simulink model "modulators"  (R2014a)
settings: Solver=ode1  StartTime=0.0  StopTime=Tsim  FixedStep=Ts  RelTol=1e-3
InitFcn:
  | GlobalParam;
undefined symbols (not defined in the file): fm, nc, tetaa, tetab, tetac, Tm, vcrls, Vs, we
libraries: simulink x36
settings Model: Creator=Leocompa  LastModifiedBy=Leocompa

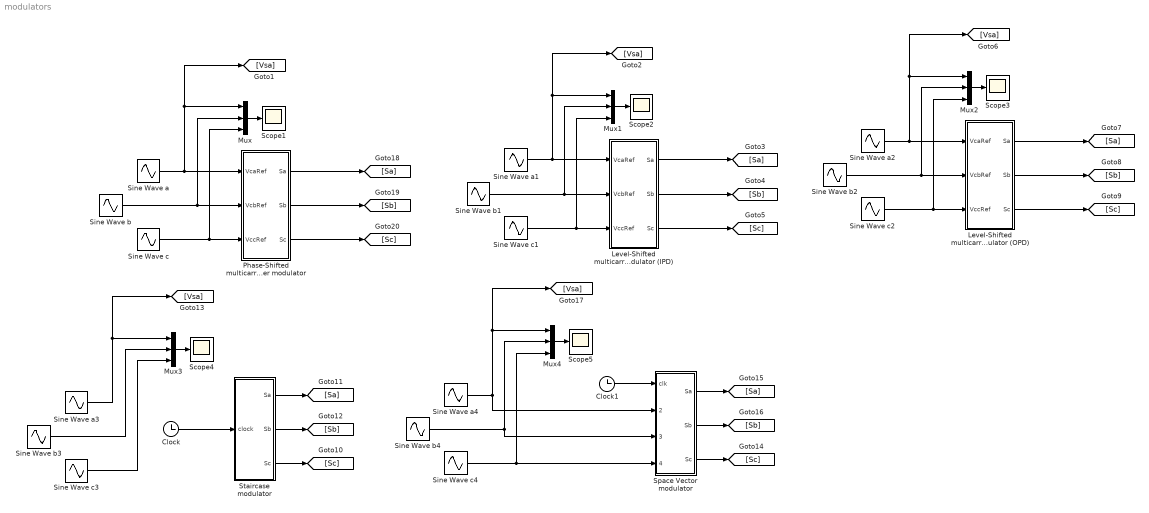
== system modulators ==
  Clock : Clock
  Clock1 : Clock
  Level-Shifted multicarrier modulator (IPD) : Subsystem
  Level-Shifted multicarrier modulator (OPD) : Subsystem
  Mux{,1..4} (5 alike) : Mux  Inputs=3
  Phase-Shifted multicarrier modulator : Subsystem
  Scope{1..5} (5 alike) : Scope
      Scope1 settings: YMin=-2500  YMax=37500  SaveName=vca1
      Scope2 settings: YMin=-2500  YMax=37500  SaveName=vca
      Scope3 settings: YMin=-2500  YMax=37500  SaveName=vca2
      Scope4 settings: YMin=-2500  YMax=37500  SaveName=vca3
      Scope5 settings: YMin=-2500  YMax=37500  SaveName=vca4
  Sine Wave a : Sin  Amplitude=Vs  Frequency=we  Phase=tetaa  SampleTime=0
  Sine Wave a1 : Sin  Amplitude=Vs  Frequency=we  SampleTime=0
  Sine Wave a2 : Sin  Amplitude=Vs  Frequency=we  SampleTime=0
  Sine Wave a3 : Sin  Amplitude=Vs  Frequency=we  Phase=tetaa  SampleTime=0
  Sine Wave a4 : Sin  Amplitude=Vs  Frequency=we  Phase=tetaa  SampleTime=0
  Sine Wave b{,1..4} (5 alike) : Sin  Amplitude=Vs  Frequency=we  Phase=tetab*pi/180  SampleTime=0
  Sine Wave c{,1..4} (5 alike) : Sin  Amplitude=Vs  Frequency=we  Phase=tetac*pi/180  SampleTime=0
  Space Vector modulator : Subsystem
  Staircase modulator : Subsystem
  wires:
  Phase-Shifted multicarrier modulator/1(Sa) -> [Sa]
  Phase-Shifted multicarrier modulator/2(Sb) -> [Sb]
  Phase-Shifted multicarrier modulator/3(Sc) -> [Sc]
  Sine Wave a/1 -> [Vsa], Mux/1, Phase-Shifted multicarrier modulator/1(VcaRef)
  Sine Wave b/1 -> Mux/2, Phase-Shifted multicarrier modulator/2(VcbRef)
  Sine Wave c/1 -> Mux/3, Phase-Shifted multicarrier modulator/3(VccRef)
  Mux/1 -> Scope1/1
  Level-Shifted multicarrier modulator (IPD)/1(Sa) -> [Sa]
  Level-Shifted multicarrier modulator (IPD)/2(Sb) -> [Sb]
  Level-Shifted multicarrier modulator (IPD)/3(Sc) -> [Sc]
  Sine Wave a1/1 -> [Vsa], Mux1/1, Level-Shifted multicarrier modulator (IPD)/1(VcaRef)
  Sine Wave b1/1 -> Mux1/2, Level-Shifted multicarrier modulator (IPD)/2(VcbRef)
  Sine Wave c1/1 -> Mux1/3, Level-Shifted multicarrier modulator (IPD)/3(VccRef)
  Mux1/1 -> Scope2/1
  Level-Shifted multicarrier modulator (OPD)/1(Sa) -> [Sa]
  Level-Shifted multicarrier modulator (OPD)/2(Sb) -> [Sb]
  Level-Shifted multicarrier modulator (OPD)/3(Sc) -> [Sc]
  Sine Wave a2/1 -> [Vsa], Mux2/1, Level-Shifted multicarrier modulator (OPD)/1(VcaRef)
  Sine Wave b2/1 -> Mux2/2, Level-Shifted multicarrier modulator (OPD)/2(VcbRef)
  Sine Wave c2/1 -> Mux2/3, Level-Shifted multicarrier modulator (OPD)/3(VccRef)
  Mux2/1 -> Scope3/1
  Sine Wave a3/1 -> [Vsa], Mux3/1
  Sine Wave b3/1 -> Mux3/2
  Sine Wave c3/1 -> Mux3/3
  Mux3/1 -> Scope4/1
  Clock/1 -> Staircase modulator/1(clock)
  Staircase modulator/3(Sc) -> [Sc]
  Staircase modulator/2(Sb) -> [Sb]
  Staircase modulator/1(Sa) -> [Sa]
  Sine Wave a4/1 -> Space Vector modulator/2(vca ref), [Vsa], Mux4/1
  Sine Wave b4/1 -> Mux4/2, Space Vector modulator/3(vcb ref1)
  Sine Wave c4/1 -> Mux4/3, Space Vector modulator/4(vcc ref2)
  Mux4/1 -> Scope5/1
  Clock1/1 -> Space Vector modulator/1(clk)
  Space Vector modulator/3(Sc) -> [Sc]
  Space Vector modulator/2(Sb) -> [Sb]
  Space Vector modulator/1(Sa) -> [Sa]

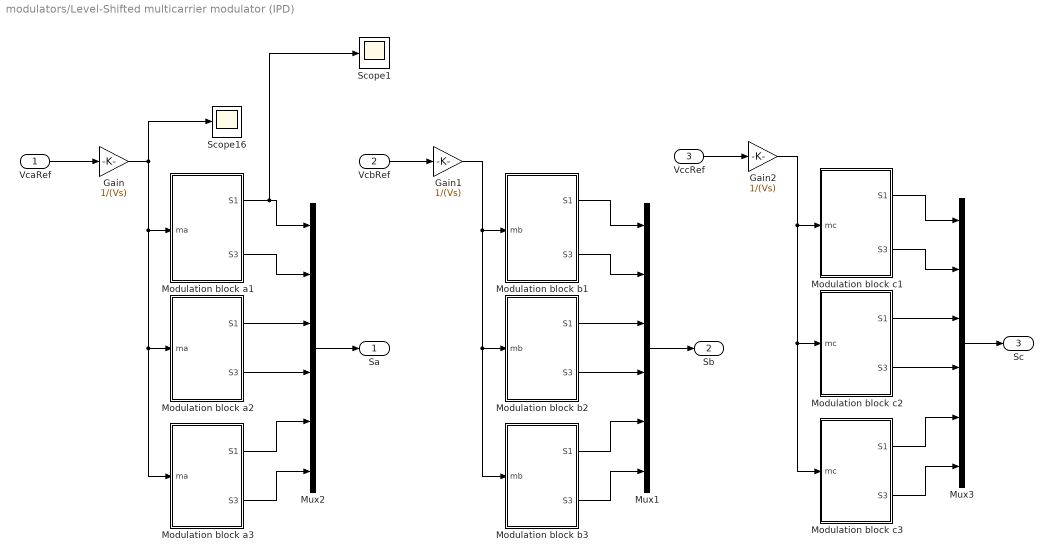
== system modulators/Level-Shifted multicarrier modulator (IPD) ==
  VcaRef : Inport
  VcbRef : Inport  Port=2
  VccRef : Inport  Port=3
  Gain : Gain  Gain=1/(Vs)
  Gain1 : Gain  Gain=1/(Vs)
  Gain2 : Gain  Gain=1/(Vs)
  Modulation block a1 : Subsystem
  Modulation block a2 : Subsystem
  Modulation block a3 : Subsystem
  Modulation block b1 : Subsystem
  Modulation block b2 : Subsystem
  Modulation block b3 : Subsystem
  Modulation block c1 : Subsystem
  Modulation block c2 : Subsystem
  Modulation block c3 : Subsystem
  Mux1 : Mux  Inputs=6
  Mux2 : Mux  Inputs=6
  Mux3 : Mux  Inputs=6
  Scope1 : Scope
      settings: SaveName=vg11
  Scope16 : Scope
      settings: YMin=-1  YMax=0.7  SaveName=vcareftri
  Sa : Outport
  Sb : Outport  Port=2
  Sc : Outport  Port=3
  wires:
  Gain/1 -> Modulation block a1/1(ma), Modulation block a3/1(ma), Modulation block a2/1(ma), Scope16/1
  Modulation block a2/2(S3) -> Mux2/4
  Modulation block a2/1(S1) -> Mux2/3
  Modulation block a3/1(S1) -> Mux2/5
  Modulation block a3/2(S3) -> Mux2/6
  Modulation block a1/2(S3) -> Mux2/2
  Modulation block a1/1(S1) -> Scope1/1, Mux2/1
  Mux2/1 -> Sa/1
  VcaRef/1 -> Gain/1
  Gain1/1 -> Modulation block b1/1(mb), Modulation block b3/1(mb), Modulation block b2/1(mb)
  Modulation block b2/2(S3) -> Mux1/4
  Modulation block b2/1(S1) -> Mux1/3
  Modulation block b3/1(S1) -> Mux1/5
  Modulation block b3/2(S3) -> Mux1/6
  Modulation block b1/2(S3) -> Mux1/2
  Modulation block b1/1(S1) -> Mux1/1
  Mux1/1 -> Sb/1
  VcbRef/1 -> Gain1/1
  Gain2/1 -> Modulation block c1/1(mc), Modulation block c3/1(mc), Modulation block c2/1(mc)
  Modulation block c2/2(S3) -> Mux3/4
  Modulation block c2/1(S1) -> Mux3/3
  Modulation block c3/1(S1) -> Mux3/5
  Modulation block c3/2(S3) -> Mux3/6
  Modulation block c1/2(S3) -> Mux3/2
  Modulation block c1/1(S1) -> Mux3/1
  Mux3/1 -> Sc/1
  VccRef/1 -> Gain2/1

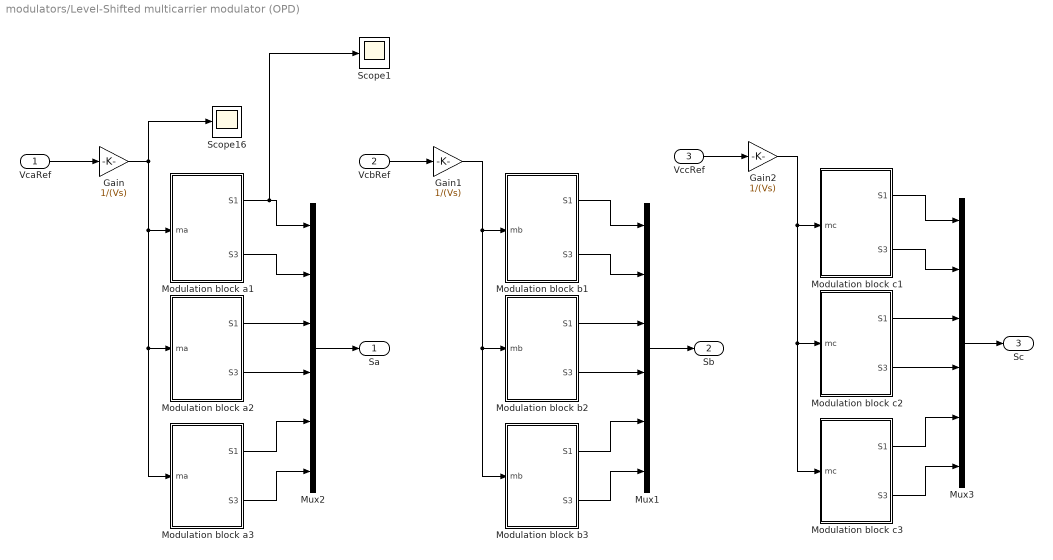
== system modulators/Level-Shifted multicarrier modulator (OPD) ==
  VcaRef : Inport
  VcbRef : Inport  Port=2
  VccRef : Inport  Port=3
  Gain : Gain  Gain=1/(Vs)
  Gain1 : Gain  Gain=1/(Vs)
  Gain2 : Gain  Gain=1/(Vs)
  Modulation block a1 : Subsystem
  Modulation block a2 : Subsystem
  Modulation block a3 : Subsystem
  Modulation block b1 : Subsystem
  Modulation block b2 : Subsystem
  Modulation block b3 : Subsystem
  Modulation block c1 : Subsystem
  Modulation block c2 : Subsystem
  Modulation block c3 : Subsystem
  Mux1 : Mux  Inputs=6
  Mux2 : Mux  Inputs=6
  Mux3 : Mux  Inputs=6
  Scope1 : Scope
      settings: SaveName=vg11
  Scope16 : Scope
      settings: YMin=-1  YMax=0.7  SaveName=vcareftri
  Sa : Outport
  Sb : Outport  Port=2
  Sc : Outport  Port=3
  wires:
  Gain/1 -> Modulation block a1/1(ma), Modulation block a3/1(ma), Modulation block a2/1(ma), Scope16/1
  Modulation block a2/2(S3) -> Mux2/4
  Modulation block a2/1(S1) -> Mux2/3
  Modulation block a3/1(S1) -> Mux2/5
  Modulation block a3/2(S3) -> Mux2/6
  Modulation block a1/2(S3) -> Mux2/2
  Modulation block a1/1(S1) -> Scope1/1, Mux2/1
  Mux2/1 -> Sa/1
  VcaRef/1 -> Gain/1
  Gain1/1 -> Modulation block b1/1(mb), Modulation block b3/1(mb), Modulation block b2/1(mb)
  Modulation block b2/2(S3) -> Mux1/4
  Modulation block b2/1(S1) -> Mux1/3
  Modulation block b3/1(S1) -> Mux1/5
  Modulation block b3/2(S3) -> Mux1/6
  Modulation block b1/2(S3) -> Mux1/2
  Modulation block b1/1(S1) -> Mux1/1
  Mux1/1 -> Sb/1
  VcbRef/1 -> Gain1/1
  Gain2/1 -> Modulation block c1/1(mc), Modulation block c3/1(mc), Modulation block c2/1(mc)
  Modulation block c2/2(S3) -> Mux3/4
  Modulation block c2/1(S1) -> Mux3/3
  Modulation block c3/1(S1) -> Mux3/5
  Modulation block c3/2(S3) -> Mux3/6
  Modulation block c1/2(S3) -> Mux3/2
  Modulation block c1/1(S1) -> Mux3/1
  Mux3/1 -> Sc/1
  VccRef/1 -> Gain2/1

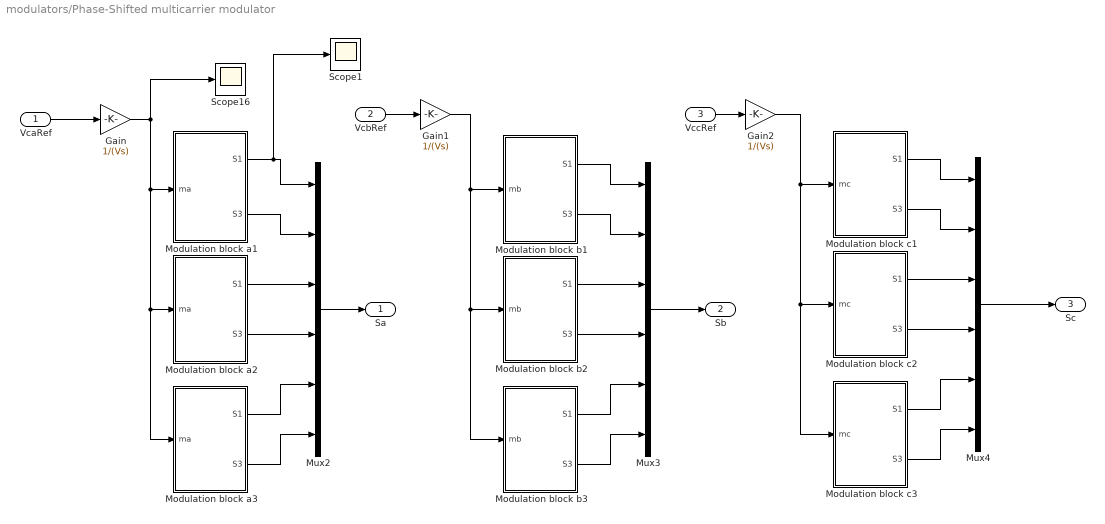
== system modulators/Phase-Shifted multicarrier modulator ==
  VcaRef : Inport
  VcbRef : Inport  Port=2
  VccRef : Inport  Port=3
  Gain : Gain  Gain=1/(Vs)
  Gain1 : Gain  Gain=1/(Vs)
  Gain2 : Gain  Gain=1/(Vs)
  Modulation block a1 : Subsystem
  Modulation block a2 : Subsystem
  Modulation block a3 : Subsystem
  Modulation block b1 : Subsystem
  Modulation block b2 : Subsystem
  Modulation block b3 : Subsystem
  Modulation block c1 : Subsystem
  Modulation block c2 : Subsystem
  Modulation block c3 : Subsystem
  Mux2 : Mux  Inputs=6
  Mux3 : Mux  Inputs=6
  Mux4 : Mux  Inputs=6
  Scope1 : Scope
      settings: SaveName=vg11
  Scope16 : Scope
      settings: YMin=-1  YMax=0.7  SaveName=vcareftri
  Sa : Outport
  Sb : Outport  Port=2
  Sc : Outport  Port=3
  wires:
  Gain1/1 -> Modulation block b1/1(mb), Modulation block b2/1(mb), Modulation block b3/1(mb)
  Gain2/1 -> Modulation block c1/1(mc), Modulation block c2/1(mc), Modulation block c3/1(mc)
  Gain/1 -> Modulation block a1/1(ma), Modulation block a3/1(ma), Modulation block a2/1(ma), Scope16/1
  Modulation block a2/2(S3) -> Mux2/4
  Modulation block a2/1(S1) -> Mux2/3
  Modulation block a3/1(S1) -> Mux2/5
  Modulation block a3/2(S3) -> Mux2/6
  Modulation block a1/2(S3) -> Mux2/2
  Mux2/1 -> Sa/1
  Modulation block b2/2(S3) -> Mux3/4
  Modulation block b3/1(S1) -> Mux3/5
  Modulation block b3/2(S3) -> Mux3/6
  Modulation block b2/1(S1) -> Mux3/3
  Modulation block b1/2(S3) -> Mux3/2
  Modulation block b1/1(S1) -> Mux3/1
  Modulation block c3/1(S1) -> Mux4/5
  Modulation block c2/1(S1) -> Mux4/3
  Modulation block c2/2(S3) -> Mux4/4
  Mux4/1 -> Sc/1
  Modulation block c1/2(S3) -> Mux4/2
  Modulation block c1/1(S1) -> Mux4/1
  Modulation block c3/2(S3) -> Mux4/6
  Mux3/1 -> Sb/1
  VcbRef/1 -> Gain1/1
  VccRef/1 -> Gain2/1
  VcaRef/1 -> Gain/1
  Modulation block a1/1(S1) -> Scope1/1, Mux2/1

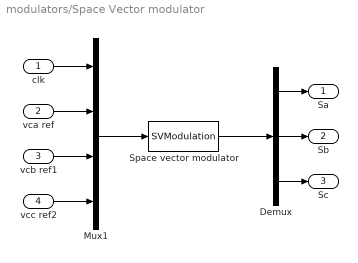
== system modulators/Space Vector modulator ==
  clk : Inport
  vca ref : Inport  Port=2
  vcb ref1 : Inport  Port=3
  vcc ref2 : Inport  Port=4
  Demux : Demux  Outputs=3
  Mux1 : Mux
  Space vector modulator : MATLABFcn  MATLABFcn=SVModulation
  Sa : Outport
  Sb : Outport  Port=2
  Sc : Outport  Port=3
  wires:
  vcc ref2/1 -> Mux1/4
  vcb ref1/1 -> Mux1/3
  vca ref/1 -> Mux1/2
  clk/1 -> Mux1/1
  Mux1/1 -> Space vector modulator/1
  Demux/3 -> Sc/1
  Demux/2 -> Sb/1
  Demux/1 -> Sa/1
  Space vector modulator/1 -> Demux/1

== system modulators/Staircase modulator ==
  clock : Inport
  Staircase modulator per phase : MATLABFcn  MATLABFcn=Staircase
  Transport Delay : TransportDelay  DelayTime=Tm*(tetab)/360
  Transport Delay1 : TransportDelay  DelayTime=Tm*(tetac)/360
  Sa : Outport
  Sb : Outport  Port=2
  Sc : Outport  Port=3
  wires:
  Transport Delay1/1 -> Sc/1
  Staircase modulator per phase/1 -> Sa/1, Transport Delay1/1, Transport Delay/1
  clock/1 -> Staircase modulator per phase/1
  Transport Delay/1 -> Sb/1

== system modulators/Level-Shifted multicarrier modulator (IPD)/Modulation block a1 ==
  ma : Inport
  Data Type Conversion : DataTypeConversion  OutDataTypeStr=double
  Data Type Conversion3 : DataTypeConversion  OutDataTypeStr=double
  Relational Operator : RelationalOperator  Operator=<=  OutDataTypeStr=boolean
  Relational Operator2 : RelationalOperator  Operator=<=  OutDataTypeStr=boolean
  Repeating Sequence1 : simulink/Sources/Repeating Sequence  rep_seq_t="[0 (1/fm)/2  1/fm]"  rep_seq_y=[4*vcrls 6*vcrls 4*vcrls]
  Repeating Sequence2 : simulink/Sources/Repeating Sequence  rep_seq_t="[0 (1/fm)/2  1/fm]"  rep_seq_y=[-6*vcrls -4*vcrls -6*vcrls]
  S1 : Outport
  S3 : Outport  Port=2
  wires:
  Relational Operator/1 -> Data Type Conversion/1
  Data Type Conversion/1 -> S1/1
  Relational Operator2/1 -> Data Type Conversion3/1
  Data Type Conversion3/1 -> S3/1
  ma/1 -> Relational Operator/2, Relational Operator2/1
  Repeating Sequence1/1 -> Relational Operator/1
  Repeating Sequence2/1 -> Relational Operator2/2

== system modulators/Level-Shifted multicarrier modulator (IPD)/Modulation block a2 ==
  ma : Inport
  Data Type Conversion : DataTypeConversion  OutDataTypeStr=double
  Data Type Conversion3 : DataTypeConversion  OutDataTypeStr=double
  Relational Operator : RelationalOperator  Operator=<=  OutDataTypeStr=boolean
  Relational Operator2 : RelationalOperator  Operator=<=  OutDataTypeStr=boolean
  Repeating Sequence1 : simulink/Sources/Repeating Sequence  rep_seq_t="[0 (1/fm)/2  1/fm]"  rep_seq_y=[2*vcrls 4*vcrls 2*vcrls]
  Repeating Sequence2 : simulink/Sources/Repeating Sequence  rep_seq_t="[0 (1/fm)/2  1/fm]"  rep_seq_y=[-4*vcrls -2*vcrls -4*vcrls]
  S1 : Outport
  S3 : Outport  Port=2
  wires:
  Relational Operator/1 -> Data Type Conversion/1
  Data Type Conversion/1 -> S1/1
  Relational Operator2/1 -> Data Type Conversion3/1
  Data Type Conversion3/1 -> S3/1
  ma/1 -> Relational Operator2/1, Relational Operator/2
  Repeating Sequence1/1 -> Relational Operator/1
  Repeating Sequence2/1 -> Relational Operator2/2

== system modulators/Level-Shifted multicarrier modulator (IPD)/Modulation block a3 ==
  ma : Inport
  Data Type Conversion : DataTypeConversion  OutDataTypeStr=double
  Data Type Conversion3 : DataTypeConversion  OutDataTypeStr=double
  Relational Operator : RelationalOperator  Operator=<=  OutDataTypeStr=boolean
  Relational Operator2 : RelationalOperator  Operator=<=  OutDataTypeStr=boolean
  Repeating Sequence1 : simulink/Sources/Repeating Sequence  rep_seq_t="[0 (1/fm)/2  1/fm]"  rep_seq_y=[0*vcrls 2*vcrls 0*vcrls]
  Repeating Sequence2 : simulink/Sources/Repeating Sequence  rep_seq_t="[0 (1/fm)/2  1/fm]"  rep_seq_y=[-2*vcrls 0 -2*vcrls]
  S1 : Outport
  S3 : Outport  Port=2
  wires:
  Relational Operator/1 -> Data Type Conversion/1
  Data Type Conversion/1 -> S1/1
  Relational Operator2/1 -> Data Type Conversion3/1
  Data Type Conversion3/1 -> S3/1
  ma/1 -> Relational Operator2/1, Relational Operator/2
  Repeating Sequence1/1 -> Relational Operator/1
  Repeating Sequence2/1 -> Relational Operator2/2

== system modulators/Level-Shifted multicarrier modulator (IPD)/Modulation block b1 ==
  mb : Inport
  Data Type Conversion : DataTypeConversion  OutDataTypeStr=double
  Data Type Conversion3 : DataTypeConversion  OutDataTypeStr=double
  Relational Operator : RelationalOperator  Operator=<=  OutDataTypeStr=boolean
  Relational Operator2 : RelationalOperator  Operator=<=  OutDataTypeStr=boolean
  Repeating Sequence1 : simulink/Sources/Repeating Sequence  rep_seq_t="[0 (1/fm)/2  1/fm]"  rep_seq_y=[4*vcrls 6*vcrls 4*vcrls]
  Repeating Sequence2 : simulink/Sources/Repeating Sequence  rep_seq_t="[0 (1/fm)/2  1/fm]"  rep_seq_y=[-6*vcrls -4*vcrls -6*vcrls]
  S1 : Outport
  S3 : Outport  Port=2
  wires:
  Relational Operator/1 -> Data Type Conversion/1
  Data Type Conversion/1 -> S1/1
  Relational Operator2/1 -> Data Type Conversion3/1
  Data Type Conversion3/1 -> S3/1
  mb/1 -> Relational Operator/2, Relational Operator2/1
  Repeating Sequence1/1 -> Relational Operator/1
  Repeating Sequence2/1 -> Relational Operator2/2

== system modulators/Level-Shifted multicarrier modulator (IPD)/Modulation block b2 ==
  mb : Inport
  Data Type Conversion : DataTypeConversion  OutDataTypeStr=double
  Data Type Conversion3 : DataTypeConversion  OutDataTypeStr=double
  Relational Operator : RelationalOperator  Operator=<=  OutDataTypeStr=boolean
  Relational Operator2 : RelationalOperator  Operator=<=  OutDataTypeStr=boolean
  Repeating Sequence1 : simulink/Sources/Repeating Sequence  rep_seq_t="[0 (1/fm)/2  1/fm]"  rep_seq_y=[2*vcrls 4*vcrls 2*vcrls]
  Repeating Sequence2 : simulink/Sources/Repeating Sequence  rep_seq_t="[0 (1/fm)/2  1/fm]"  rep_seq_y=[-4*vcrls -2*vcrls -4*vcrls]
  S1 : Outport
  S3 : Outport  Port=2
  wires:
  Relational Operator/1 -> Data Type Conversion/1
  Data Type Conversion/1 -> S1/1
  Relational Operator2/1 -> Data Type Conversion3/1
  Data Type Conversion3/1 -> S3/1
  mb/1 -> Relational Operator2/1, Relational Operator/2
  Repeating Sequence1/1 -> Relational Operator/1
  Repeating Sequence2/1 -> Relational Operator2/2

== system modulators/Level-Shifted multicarrier modulator (IPD)/Modulation block b3 ==
  mb : Inport
  Data Type Conversion : DataTypeConversion  OutDataTypeStr=double
  Data Type Conversion3 : DataTypeConversion  OutDataTypeStr=double
  Relational Operator : RelationalOperator  Operator=<=  OutDataTypeStr=boolean
  Relational Operator2 : RelationalOperator  Operator=<=  OutDataTypeStr=boolean
  Repeating Sequence1 : simulink/Sources/Repeating Sequence  rep_seq_t="[0 (1/fm)/2  1/fm]"  rep_seq_y=[0*vcrls 2*vcrls 0*vcrls]
  Repeating Sequence2 : simulink/Sources/Repeating Sequence  rep_seq_t="[0 (1/fm)/2  1/fm]"  rep_seq_y=[-2*vcrls 0 -2*vcrls]
  S1 : Outport
  S3 : Outport  Port=2
  wires:
  Relational Operator/1 -> Data Type Conversion/1
  Data Type Conversion/1 -> S1/1
  Relational Operator2/1 -> Data Type Conversion3/1
  Data Type Conversion3/1 -> S3/1
  mb/1 -> Relational Operator2/1, Relational Operator/2
  Repeating Sequence1/1 -> Relational Operator/1
  Repeating Sequence2/1 -> Relational Operator2/2

== system modulators/Level-Shifted multicarrier modulator (IPD)/Modulation block c1 ==
  mc : Inport
  Data Type Conversion : DataTypeConversion  OutDataTypeStr=double
  Data Type Conversion3 : DataTypeConversion  OutDataTypeStr=double
  Relational Operator : RelationalOperator  Operator=<=  OutDataTypeStr=boolean
  Relational Operator2 : RelationalOperator  Operator=<=  OutDataTypeStr=boolean
  Repeating Sequence1 : simulink/Sources/Repeating Sequence  rep_seq_t="[0 (1/fm)/2  1/fm]"  rep_seq_y=[4*vcrls 6*vcrls 4*vcrls]
  Repeating Sequence2 : simulink/Sources/Repeating Sequence  rep_seq_t="[0 (1/fm)/2  1/fm]"  rep_seq_y=[-6*vcrls -4*vcrls -6*vcrls]
  S1 : Outport
  S3 : Outport  Port=2
  wires:
  Relational Operator/1 -> Data Type Conversion/1
  Data Type Conversion/1 -> S1/1
  Relational Operator2/1 -> Data Type Conversion3/1
  Data Type Conversion3/1 -> S3/1
  mc/1 -> Relational Operator/2, Relational Operator2/1
  Repeating Sequence1/1 -> Relational Operator/1
  Repeating Sequence2/1 -> Relational Operator2/2

== system modulators/Level-Shifted multicarrier modulator (IPD)/Modulation block c2 ==
  mc : Inport
  Data Type Conversion : DataTypeConversion  OutDataTypeStr=double
  Data Type Conversion3 : DataTypeConversion  OutDataTypeStr=double
  Relational Operator : RelationalOperator  Operator=<=  OutDataTypeStr=boolean
  Relational Operator2 : RelationalOperator  Operator=<=  OutDataTypeStr=boolean
  Repeating Sequence1 : simulink/Sources/Repeating Sequence  rep_seq_t="[0 (1/fm)/2  1/fm]"  rep_seq_y=[2*vcrls 4*vcrls 2*vcrls]
  Repeating Sequence2 : simulink/Sources/Repeating Sequence  rep_seq_t="[0 (1/fm)/2  1/fm]"  rep_seq_y=[-4*vcrls -2*vcrls -4*vcrls]
  S1 : Outport
  S3 : Outport  Port=2
  wires:
  Relational Operator/1 -> Data Type Conversion/1
  Data Type Conversion/1 -> S1/1
  Relational Operator2/1 -> Data Type Conversion3/1
  Data Type Conversion3/1 -> S3/1
  mc/1 -> Relational Operator2/1, Relational Operator/2
  Repeating Sequence1/1 -> Relational Operator/1
  Repeating Sequence2/1 -> Relational Operator2/2

== system modulators/Level-Shifted multicarrier modulator (IPD)/Modulation block c3 ==
  mc : Inport
  Data Type Conversion : DataTypeConversion  OutDataTypeStr=double
  Data Type Conversion3 : DataTypeConversion  OutDataTypeStr=double
  Relational Operator : RelationalOperator  Operator=<=  OutDataTypeStr=boolean
  Relational Operator2 : RelationalOperator  Operator=<=  OutDataTypeStr=boolean
  Repeating Sequence1 : simulink/Sources/Repeating Sequence  rep_seq_t="[0 (1/fm)/2  1/fm]"  rep_seq_y=[0*vcrls 2*vcrls 0*vcrls]
  Repeating Sequence2 : simulink/Sources/Repeating Sequence  rep_seq_t="[0 (1/fm)/2  1/fm]"  rep_seq_y=[-2*vcrls 0 -2*vcrls]
  S1 : Outport
  S3 : Outport  Port=2
  wires:
  Relational Operator/1 -> Data Type Conversion/1
  Data Type Conversion/1 -> S1/1
  Relational Operator2/1 -> Data Type Conversion3/1
  Data Type Conversion3/1 -> S3/1
  mc/1 -> Relational Operator2/1, Relational Operator/2
  Repeating Sequence1/1 -> Relational Operator/1
  Repeating Sequence2/1 -> Relational Operator2/2

== system modulators/Level-Shifted multicarrier modulator (OPD)/Modulation block a1 ==
  ma : Inport
  Data Type Conversion : DataTypeConversion  OutDataTypeStr=double
  Data Type Conversion3 : DataTypeConversion  OutDataTypeStr=double
  Gain : Gain  Gain=-1
  Relational Operator : RelationalOperator  Operator=<=  OutDataTypeStr=boolean
  Relational Operator2 : RelationalOperator  Operator=<=  OutDataTypeStr=boolean
  Repeating Sequence1 : simulink/Sources/Repeating Sequence  rep_seq_t="[0 (1/fm)/2  1/fm]"  rep_seq_y=[4*vcrls 6*vcrls 4*vcrls]
  S1 : Outport
  S3 : Outport  Port=2
  wires:
  Relational Operator/1 -> Data Type Conversion/1
  Data Type Conversion/1 -> S1/1
  Relational Operator2/1 -> Data Type Conversion3/1
  Data Type Conversion3/1 -> S3/1
  ma/1 -> Relational Operator/2, Relational Operator2/1
  Repeating Sequence1/1 -> Gain/1, Relational Operator/1
  Gain/1 -> Relational Operator2/2

== system modulators/Level-Shifted multicarrier modulator (OPD)/Modulation block a2 ==
  ma : Inport
  Data Type Conversion : DataTypeConversion  OutDataTypeStr=double
  Data Type Conversion3 : DataTypeConversion  OutDataTypeStr=double
  Gain : Gain  Gain=-1
  Relational Operator : RelationalOperator  Operator=<=  OutDataTypeStr=boolean
  Relational Operator2 : RelationalOperator  Operator=<=  OutDataTypeStr=boolean
  Repeating Sequence1 : simulink/Sources/Repeating Sequence  rep_seq_t="[0 (1/fm)/2  1/fm]"  rep_seq_y=[2*vcrls 4*vcrls 2*vcrls]
  S1 : Outport
  S3 : Outport  Port=2
  wires:
  Relational Operator/1 -> Data Type Conversion/1
  Data Type Conversion/1 -> S1/1
  Relational Operator2/1 -> Data Type Conversion3/1
  Data Type Conversion3/1 -> S3/1
  ma/1 -> Relational Operator2/1, Relational Operator/2
  Repeating Sequence1/1 -> Gain/1, Relational Operator/1
  Gain/1 -> Relational Operator2/2

== system modulators/Level-Shifted multicarrier modulator (OPD)/Modulation block a3 ==
  ma : Inport
  Data Type Conversion : DataTypeConversion  OutDataTypeStr=double
  Data Type Conversion3 : DataTypeConversion  OutDataTypeStr=double
  Gain : Gain  Gain=-1
  Relational Operator : RelationalOperator  Operator=<=  OutDataTypeStr=boolean
  Relational Operator2 : RelationalOperator  Operator=<=  OutDataTypeStr=boolean
  Repeating Sequence1 : simulink/Sources/Repeating Sequence  rep_seq_t="[0 (1/fm)/2  1/fm]"  rep_seq_y=[0*vcrls 2*vcrls 0*vcrls]
  S1 : Outport
  S3 : Outport  Port=2
  wires:
  Relational Operator/1 -> Data Type Conversion/1
  Data Type Conversion/1 -> S1/1
  Relational Operator2/1 -> Data Type Conversion3/1
  Data Type Conversion3/1 -> S3/1
  ma/1 -> Relational Operator2/1, Relational Operator/2
  Gain/1 -> Relational Operator2/2
  Repeating Sequence1/1 -> Gain/1, Relational Operator/1

== system modulators/Level-Shifted multicarrier modulator (OPD)/Modulation block b1 ==
  mb : Inport
  Data Type Conversion : DataTypeConversion  OutDataTypeStr=double
  Data Type Conversion3 : DataTypeConversion  OutDataTypeStr=double
  Gain : Gain  Gain=-1
  Relational Operator : RelationalOperator  Operator=<=  OutDataTypeStr=boolean
  Relational Operator2 : RelationalOperator  Operator=<=  OutDataTypeStr=boolean
  Repeating Sequence1 : simulink/Sources/Repeating Sequence  rep_seq_t="[0 (1/fm)/2  1/fm]"  rep_seq_y=[4*vcrls 6*vcrls 4*vcrls]
  S1 : Outport
  S3 : Outport  Port=2
  wires:
  Relational Operator/1 -> Data Type Conversion/1
  Data Type Conversion/1 -> S1/1
  Relational Operator2/1 -> Data Type Conversion3/1
  Data Type Conversion3/1 -> S3/1
  mb/1 -> Relational Operator/2, Relational Operator2/1
  Repeating Sequence1/1 -> Gain/1, Relational Operator/1
  Gain/1 -> Relational Operator2/2

== system modulators/Level-Shifted multicarrier modulator (OPD)/Modulation block b2 ==
  mb : Inport
  Data Type Conversion : DataTypeConversion  OutDataTypeStr=double
  Data Type Conversion3 : DataTypeConversion  OutDataTypeStr=double
  Gain : Gain  Gain=-1
  Relational Operator : RelationalOperator  Operator=<=  OutDataTypeStr=boolean
  Relational Operator2 : RelationalOperator  Operator=<=  OutDataTypeStr=boolean
  Repeating Sequence1 : simulink/Sources/Repeating Sequence  rep_seq_t="[0 (1/fm)/2  1/fm]"  rep_seq_y=[2*vcrls 4*vcrls 2*vcrls]
  S1 : Outport
  S3 : Outport  Port=2
  wires:
  Relational Operator/1 -> Data Type Conversion/1
  Data Type Conversion/1 -> S1/1
  Relational Operator2/1 -> Data Type Conversion3/1
  Data Type Conversion3/1 -> S3/1
  mb/1 -> Relational Operator2/1, Relational Operator/2
  Repeating Sequence1/1 -> Gain/1, Relational Operator/1
  Gain/1 -> Relational Operator2/2

== system modulators/Level-Shifted multicarrier modulator (OPD)/Modulation block b3 ==
  mb : Inport
  Data Type Conversion : DataTypeConversion  OutDataTypeStr=double
  Data Type Conversion3 : DataTypeConversion  OutDataTypeStr=double
  Gain : Gain  Gain=-1
  Relational Operator : RelationalOperator  Operator=<=  OutDataTypeStr=boolean
  Relational Operator2 : RelationalOperator  Operator=<=  OutDataTypeStr=boolean
  Repeating Sequence1 : simulink/Sources/Repeating Sequence  rep_seq_t="[0 (1/fm)/2  1/fm]"  rep_seq_y=[0*vcrls 2*vcrls 0*vcrls]
  S1 : Outport
  S3 : Outport  Port=2
  wires:
  Relational Operator/1 -> Data Type Conversion/1
  Data Type Conversion/1 -> S1/1
  Relational Operator2/1 -> Data Type Conversion3/1
  Data Type Conversion3/1 -> S3/1
  mb/1 -> Relational Operator2/1, Relational Operator/2
  Gain/1 -> Relational Operator2/2
  Repeating Sequence1/1 -> Gain/1, Relational Operator/1

== system modulators/Level-Shifted multicarrier modulator (OPD)/Modulation block c1 ==
  mc : Inport
  Data Type Conversion : DataTypeConversion  OutDataTypeStr=double
  Data Type Conversion3 : DataTypeConversion  OutDataTypeStr=double
  Gain : Gain  Gain=-1
  Relational Operator : RelationalOperator  Operator=<=  OutDataTypeStr=boolean
  Relational Operator2 : RelationalOperator  Operator=<=  OutDataTypeStr=boolean
  Repeating Sequence1 : simulink/Sources/Repeating Sequence  rep_seq_t="[0 (1/fm)/2  1/fm]"  rep_seq_y=[4*vcrls 6*vcrls 4*vcrls]
  S1 : Outport
  S3 : Outport  Port=2
  wires:
  Relational Operator/1 -> Data Type Conversion/1
  Data Type Conversion/1 -> S1/1
  Relational Operator2/1 -> Data Type Conversion3/1
  Data Type Conversion3/1 -> S3/1
  mc/1 -> Relational Operator/2, Relational Operator2/1
  Repeating Sequence1/1 -> Gain/1, Relational Operator/1
  Gain/1 -> Relational Operator2/2

== system modulators/Level-Shifted multicarrier modulator (OPD)/Modulation block c2 ==
  mc : Inport
  Data Type Conversion : DataTypeConversion  OutDataTypeStr=double
  Data Type Conversion3 : DataTypeConversion  OutDataTypeStr=double
  Gain : Gain  Gain=-1
  Relational Operator : RelationalOperator  Operator=<=  OutDataTypeStr=boolean
  Relational Operator2 : RelationalOperator  Operator=<=  OutDataTypeStr=boolean
  Repeating Sequence1 : simulink/Sources/Repeating Sequence  rep_seq_t="[0 (1/fm)/2  1/fm]"  rep_seq_y=[2*vcrls 4*vcrls 2*vcrls]
  S1 : Outport
  S3 : Outport  Port=2
  wires:
  Relational Operator/1 -> Data Type Conversion/1
  Data Type Conversion/1 -> S1/1
  Relational Operator2/1 -> Data Type Conversion3/1
  Data Type Conversion3/1 -> S3/1
  mc/1 -> Relational Operator2/1, Relational Operator/2
  Repeating Sequence1/1 -> Gain/1, Relational Operator/1
  Gain/1 -> Relational Operator2/2

== system modulators/Level-Shifted multicarrier modulator (OPD)/Modulation block c3 ==
  mc : Inport
  Data Type Conversion : DataTypeConversion  OutDataTypeStr=double
  Data Type Conversion3 : DataTypeConversion  OutDataTypeStr=double
  Gain : Gain  Gain=-1
  Relational Operator : RelationalOperator  Operator=<=  OutDataTypeStr=boolean
  Relational Operator2 : RelationalOperator  Operator=<=  OutDataTypeStr=boolean
  Repeating Sequence1 : simulink/Sources/Repeating Sequence  rep_seq_t="[0 (1/fm)/2  1/fm]"  rep_seq_y=[0*vcrls 2*vcrls 0*vcrls]
  S1 : Outport
  S3 : Outport  Port=2
  wires:
  Relational Operator/1 -> Data Type Conversion/1
  Data Type Conversion/1 -> S1/1
  Relational Operator2/1 -> Data Type Conversion3/1
  Data Type Conversion3/1 -> S3/1
  mc/1 -> Relational Operator2/1, Relational Operator/2
  Gain/1 -> Relational Operator2/2
  Repeating Sequence1/1 -> Gain/1, Relational Operator/1

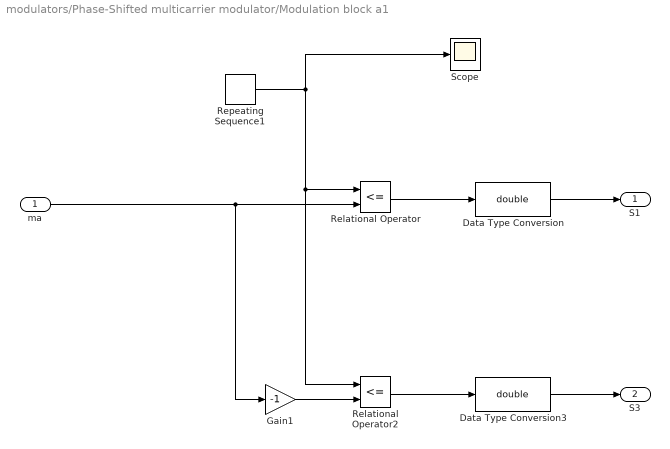
== system modulators/Phase-Shifted multicarrier modulator/Modulation block a1 ==
  ma : Inport
  Data Type Conversion : DataTypeConversion  OutDataTypeStr=double
  Data Type Conversion3 : DataTypeConversion  OutDataTypeStr=double
  Gain1 : Gain  Gain=-1
  Relational Operator : RelationalOperator  Operator=<=  OutDataTypeStr=boolean
  Relational Operator2 : RelationalOperator  Operator=<=  OutDataTypeStr=boolean
  Repeating Sequence1 : simulink/Sources/Repeating Sequence  rep_seq_t="[0 (1/fm)/2  1/fm]"  rep_seq_y=[-1 1 -1]
  Scope : Scope
      settings: SaveName=carrier
  S1 : Outport
  S3 : Outport  Port=2
  wires:
  Relational Operator/1 -> Data Type Conversion/1
  Repeating Sequence1/1 -> Scope/1, Relational Operator/1, Relational Operator2/1
  Data Type Conversion/1 -> S1/1
  ma/1 -> Relational Operator/2, Gain1/1
  Relational Operator2/1 -> Data Type Conversion3/1
  Data Type Conversion3/1 -> S3/1
  Gain1/1 -> Relational Operator2/2

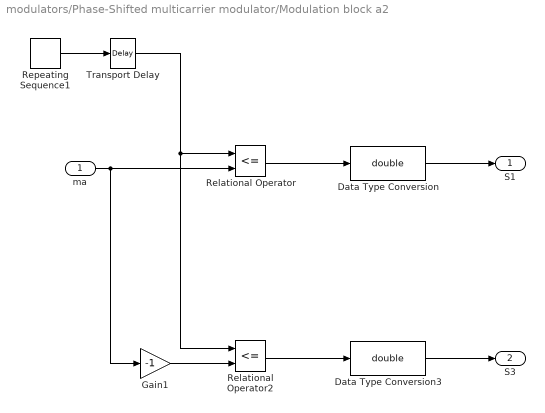
== system modulators/Phase-Shifted multicarrier modulator/Modulation block a2 ==
  ma : Inport
  Data Type Conversion : DataTypeConversion  OutDataTypeStr=double
  Data Type Conversion3 : DataTypeConversion  OutDataTypeStr=double
  Gain1 : Gain  Gain=-1
  Relational Operator : RelationalOperator  Operator=<=  OutDataTypeStr=boolean
  Relational Operator2 : RelationalOperator  Operator=<=  OutDataTypeStr=boolean
  Repeating Sequence1 : simulink/Sources/Repeating Sequence  rep_seq_t="[0 (1/fm)/2  1/fm]"  rep_seq_y=[-1 1 -1]
  Transport Delay : TransportDelay  DelayTime=Tm*(180/nc)/360
  S1 : Outport
  S3 : Outport  Port=2
  wires:
  Relational Operator/1 -> Data Type Conversion/1
  Repeating Sequence1/1 -> Transport Delay/1
  Data Type Conversion/1 -> S1/1
  ma/1 -> Relational Operator/2, Gain1/1
  Relational Operator2/1 -> Data Type Conversion3/1
  Data Type Conversion3/1 -> S3/1
  Gain1/1 -> Relational Operator2/2
  Transport Delay/1 -> Relational Operator/1, Relational Operator2/1

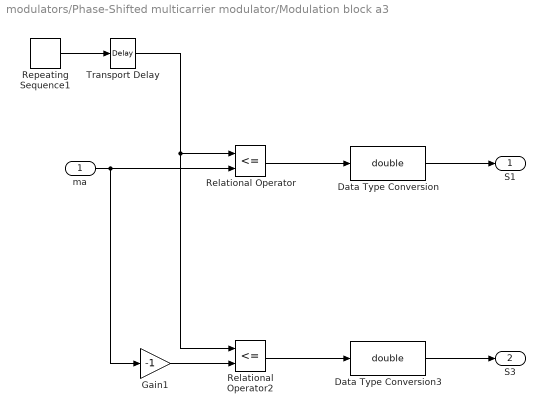
== system modulators/Phase-Shifted multicarrier modulator/Modulation block a3 ==
  ma : Inport
  Data Type Conversion : DataTypeConversion  OutDataTypeStr=double
  Data Type Conversion3 : DataTypeConversion  OutDataTypeStr=double
  Gain1 : Gain  Gain=-1
  Relational Operator : RelationalOperator  Operator=<=  OutDataTypeStr=boolean
  Relational Operator2 : RelationalOperator  Operator=<=  OutDataTypeStr=boolean
  Repeating Sequence1 : simulink/Sources/Repeating Sequence  rep_seq_t="[0 (1/fm)/2  1/fm]"  rep_seq_y=[-1 1 -1]
  Transport Delay : TransportDelay  DelayTime=(Tm*(180/nc)/360)*2
  S1 : Outport
  S3 : Outport  Port=2
  wires:
  Relational Operator/1 -> Data Type Conversion/1
  Repeating Sequence1/1 -> Transport Delay/1
  Data Type Conversion/1 -> S1/1
  ma/1 -> Relational Operator/2, Gain1/1
  Relational Operator2/1 -> Data Type Conversion3/1
  Data Type Conversion3/1 -> S3/1
  Gain1/1 -> Relational Operator2/2
  Transport Delay/1 -> Relational Operator/1, Relational Operator2/1

== system modulators/Phase-Shifted multicarrier modulator/Modulation block b1 ==
  mb : Inport
  Data Type Conversion : DataTypeConversion  OutDataTypeStr=double
  Data Type Conversion3 : DataTypeConversion  OutDataTypeStr=double
  Gain1 : Gain  Gain=-1
  Relational Operator : RelationalOperator  Operator=<=  OutDataTypeStr=boolean
  Relational Operator2 : RelationalOperator  Operator=<=  OutDataTypeStr=boolean
  Repeating Sequence1 : simulink/Sources/Repeating Sequence  rep_seq_t="[0 (1/fm)/2  1/fm]"  rep_seq_y=[-1 1 -1]
  S1 : Outport
  S3 : Outport  Port=2
  wires:
  Relational Operator/1 -> Data Type Conversion/1
  Repeating Sequence1/1 -> Relational Operator/1, Relational Operator2/1
  Data Type Conversion/1 -> S1/1
  mb/1 -> Relational Operator/2, Gain1/1
  Relational Operator2/1 -> Data Type Conversion3/1
  Data Type Conversion3/1 -> S3/1
  Gain1/1 -> Relational Operator2/2

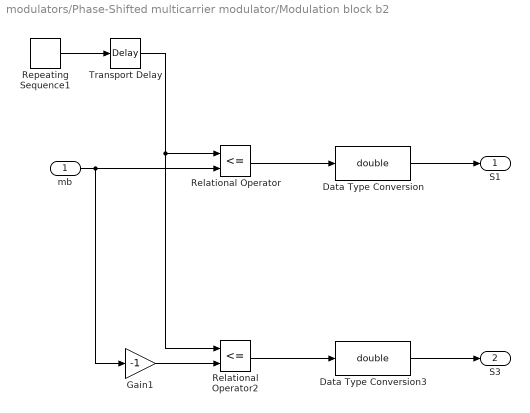
== system modulators/Phase-Shifted multicarrier modulator/Modulation block b2 ==
  mb : Inport
  Data Type Conversion : DataTypeConversion  OutDataTypeStr=double
  Data Type Conversion3 : DataTypeConversion  OutDataTypeStr=double
  Gain1 : Gain  Gain=-1
  Relational Operator : RelationalOperator  Operator=<=  OutDataTypeStr=boolean
  Relational Operator2 : RelationalOperator  Operator=<=  OutDataTypeStr=boolean
  Repeating Sequence1 : simulink/Sources/Repeating Sequence  rep_seq_t="[0 (1/fm)/2  1/fm]"  rep_seq_y=[-1 1 -1]
  Transport Delay : TransportDelay  DelayTime=Tm*(180/nc)/360
  S1 : Outport
  S3 : Outport  Port=2
  wires:
  Relational Operator/1 -> Data Type Conversion/1
  Repeating Sequence1/1 -> Transport Delay/1
  Data Type Conversion/1 -> S1/1
  mb/1 -> Relational Operator/2, Gain1/1
  Relational Operator2/1 -> Data Type Conversion3/1
  Data Type Conversion3/1 -> S3/1
  Gain1/1 -> Relational Operator2/2
  Transport Delay/1 -> Relational Operator/1, Relational Operator2/1

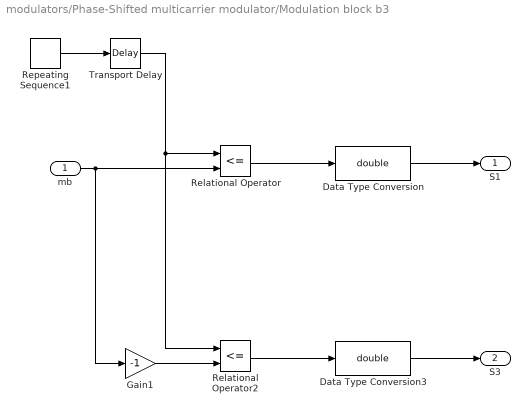
== system modulators/Phase-Shifted multicarrier modulator/Modulation block b3 ==
  mb : Inport
  Data Type Conversion : DataTypeConversion  OutDataTypeStr=double
  Data Type Conversion3 : DataTypeConversion  OutDataTypeStr=double
  Gain1 : Gain  Gain=-1
  Relational Operator : RelationalOperator  Operator=<=  OutDataTypeStr=boolean
  Relational Operator2 : RelationalOperator  Operator=<=  OutDataTypeStr=boolean
  Repeating Sequence1 : simulink/Sources/Repeating Sequence  rep_seq_t="[0 (1/fm)/2  1/fm]"  rep_seq_y=[-1 1 -1]
  Transport Delay : TransportDelay  DelayTime=(Tm*(180/nc)/360)*2
  S1 : Outport
  S3 : Outport  Port=2
  wires:
  Relational Operator/1 -> Data Type Conversion/1
  Repeating Sequence1/1 -> Transport Delay/1
  Data Type Conversion/1 -> S1/1
  mb/1 -> Relational Operator/2, Gain1/1
  Relational Operator2/1 -> Data Type Conversion3/1
  Data Type Conversion3/1 -> S3/1
  Gain1/1 -> Relational Operator2/2
  Transport Delay/1 -> Relational Operator/1, Relational Operator2/1

== system modulators/Phase-Shifted multicarrier modulator/Modulation block c1 ==
  mc : Inport
  Data Type Conversion : DataTypeConversion  OutDataTypeStr=double
  Data Type Conversion3 : DataTypeConversion  OutDataTypeStr=double
  Gain1 : Gain  Gain=-1
  Relational Operator : RelationalOperator  Operator=<=  OutDataTypeStr=boolean
  Relational Operator2 : RelationalOperator  Operator=<=  OutDataTypeStr=boolean
  Repeating Sequence1 : simulink/Sources/Repeating Sequence  rep_seq_t="[0 (1/fm)/2  1/fm]"  rep_seq_y=[-1 1 -1]
  S1 : Outport
  S3 : Outport  Port=2
  wires:
  Relational Operator/1 -> Data Type Conversion/1
  Repeating Sequence1/1 -> Relational Operator/1, Relational Operator2/1
  Data Type Conversion/1 -> S1/1
  mc/1 -> Relational Operator/2, Gain1/1
  Relational Operator2/1 -> Data Type Conversion3/1
  Data Type Conversion3/1 -> S3/1
  Gain1/1 -> Relational Operator2/2

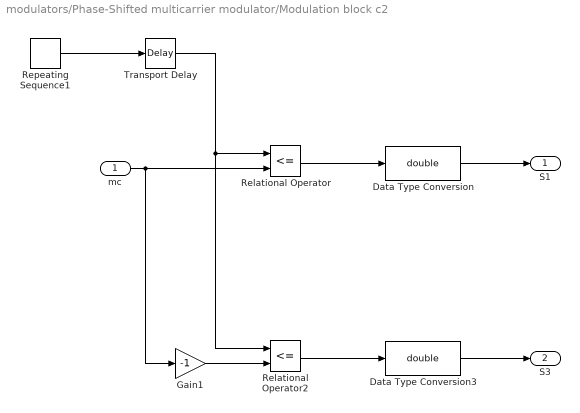
== system modulators/Phase-Shifted multicarrier modulator/Modulation block c2 ==
  mc : Inport
  Data Type Conversion : DataTypeConversion  OutDataTypeStr=double
  Data Type Conversion3 : DataTypeConversion  OutDataTypeStr=double
  Gain1 : Gain  Gain=-1
  Relational Operator : RelationalOperator  Operator=<=  OutDataTypeStr=boolean
  Relational Operator2 : RelationalOperator  Operator=<=  OutDataTypeStr=boolean
  Repeating Sequence1 : simulink/Sources/Repeating Sequence  rep_seq_t="[0 (1/fm)/2  1/fm]"  rep_seq_y=[-1 1 -1]
  Transport Delay : TransportDelay  DelayTime=(Tm*(180/nc)/360)*2
  S1 : Outport
  S3 : Outport  Port=2
  wires:
  Relational Operator/1 -> Data Type Conversion/1
  Repeating Sequence1/1 -> Transport Delay/1
  Data Type Conversion/1 -> S1/1
  mc/1 -> Relational Operator/2, Gain1/1
  Relational Operator2/1 -> Data Type Conversion3/1
  Data Type Conversion3/1 -> S3/1
  Gain1/1 -> Relational Operator2/2
  Transport Delay/1 -> Relational Operator/1, Relational Operator2/1

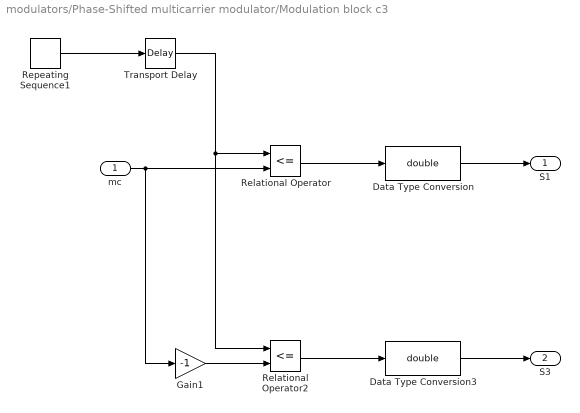
== system modulators/Phase-Shifted multicarrier modulator/Modulation block c3 ==
  mc : Inport
  Data Type Conversion : DataTypeConversion  OutDataTypeStr=double
  Data Type Conversion3 : DataTypeConversion  OutDataTypeStr=double
  Gain1 : Gain  Gain=-1
  Relational Operator : RelationalOperator  Operator=<=  OutDataTypeStr=boolean
  Relational Operator2 : RelationalOperator  Operator=<=  OutDataTypeStr=boolean
  Repeating Sequence1 : simulink/Sources/Repeating Sequence  rep_seq_t="[0 (1/fm)/2  1/fm]"  rep_seq_y=[-1 1 -1]
  Transport Delay : TransportDelay  DelayTime=(Tm*(180/nc)/360)*2
  S1 : Outport
  S3 : Outport  Port=2
  wires:
  Relational Operator/1 -> Data Type Conversion/1
  Repeating Sequence1/1 -> Transport Delay/1
  Data Type Conversion/1 -> S1/1
  mc/1 -> Relational Operator/2, Gain1/1
  Relational Operator2/1 -> Data Type Conversion3/1
  Data Type Conversion3/1 -> S3/1
  Gain1/1 -> Relational Operator2/2
  Transport Delay/1 -> Relational Operator/1, Relational Operator2/1
